simulink model "Mars_capture_sim"  (R2024b)
settings: Solver=VariableStepAuto  StartTime=0.0  StopTime=5e5  MaxStep=50  RelTol=1e-6
values from neighbouring files (symbols this model uses):
  capture_data = capture(Mars_planet,altitude,i,theta,transfer_data)    [Mars_capture_setup.m]
settings Model: Creator=cpero  LastModifiedBy=cpero

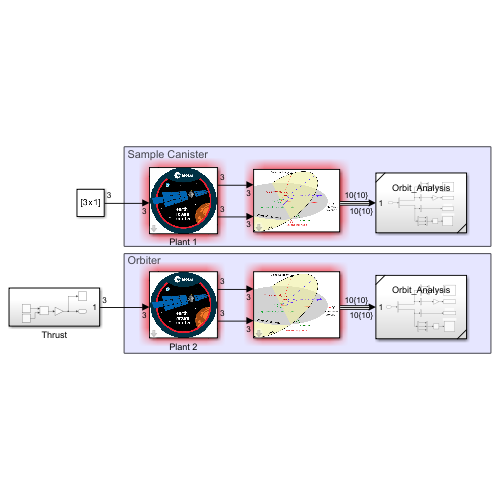
[thumbnail: Simulink's stored preview of the top-level diagram]
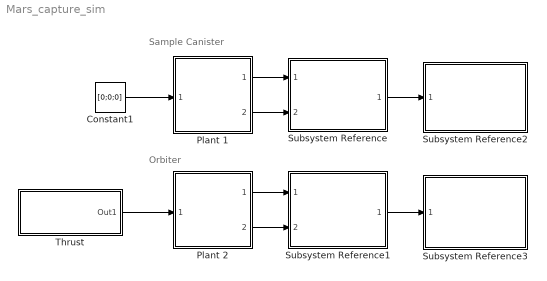
== system Mars_capture_sim ==
  note: Orbiter
  note: Sample Canister
  Constant1 : Constant  Value=[0;0;0]
  Plant 1 : Subsystem  ReferencedSubsystem=Plant  setup=capture_data.canister_initial  switch_time=0  mu=Mars_planet.mu
  Plant 2 : Subsystem  ReferencedSubsystem=Plant  setup=capture_data.orbiter_initial  switch_time=0  mu=Mars_planet.mu
  Subsystem Reference : Subsystem  ReferencedSubsystem=Orbit_Calculations  mu=Mars_planet.mu
  Subsystem Reference1 : Subsystem  ReferencedSubsystem=Orbit_Calculations  mu=Mars_planet.mu
  Subsystem Reference2 : Subsystem  ReferencedSubsystem=Orbit_Analysis
  Subsystem Reference3 : Subsystem  ReferencedSubsystem=Orbit_Analysis
  Thrust : Subsystem
  wires:
  Plant 1/1 -> Subsystem Reference/1
  Plant 2/1 -> Subsystem Reference1/1
  Plant 2/2 -> Subsystem Reference1/2
  Plant 1/2 -> Subsystem Reference/2
  Thrust/1(Out1) -> Plant 2/1
  Constant1/1 -> Plant 1/1
  Subsystem Reference/1 -> Subsystem Reference2/1
  Subsystem Reference1/1 -> Subsystem Reference3/1

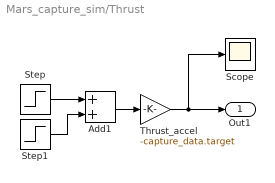
== system Mars_capture_sim/Thrust ==
  Add1 : Sum
  Scope : Scope
  Step : Step  Time=3.714e5  SampleTime=0
  Step1 : Step  Time=3.714e5 + 1  After=-1  SampleTime=0
  Thrust_accel : Gain  Gain=-capture_data.target
  Out1 : Outport
  wires:
  Add1/1 -> Thrust_accel/1
  Thrust_accel/1 -> Out1/1, Scope/1
  Step1/1 -> Add1/2
  Step/1 -> Add1/1
